simulink model "model6_3"  (R2025a)
settings: Solver=VariableStepAuto  StartTime=0.0  StopTime=100000  RelTol=1e-3
values from neighbouring files (symbols this model uses):
  Tf = 1    [domaci6_1.m]
settings Model: Creator=neso  LastModifiedBy=Nenad

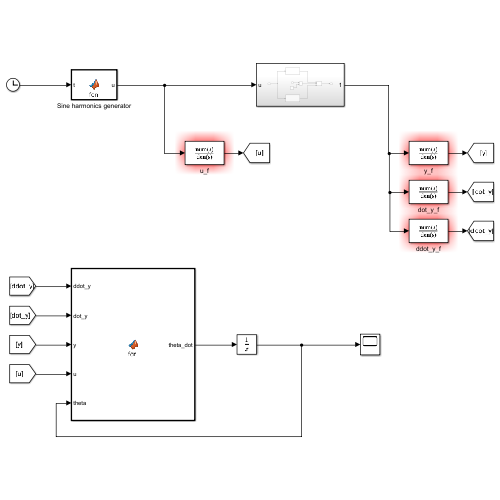
[thumbnail: Simulink's stored preview of the top-level diagram]
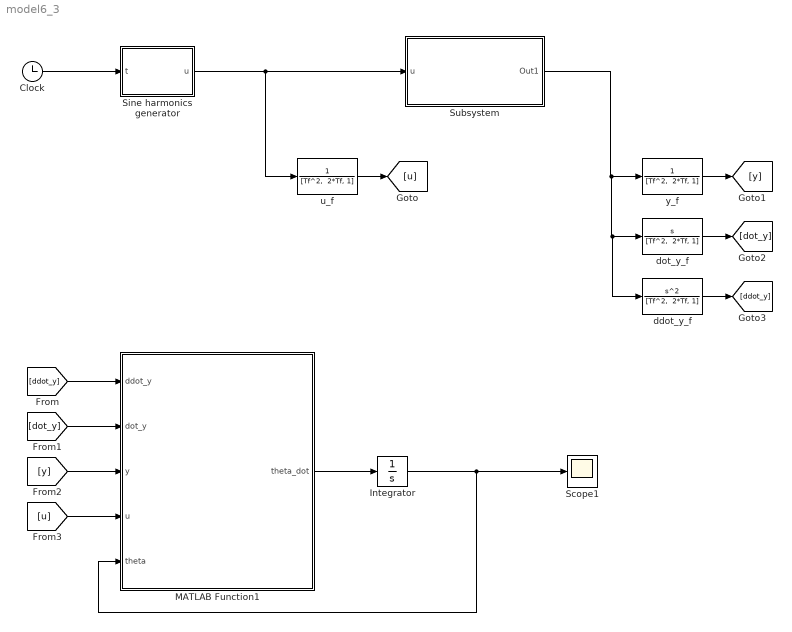
== system model6_3 ==
  Clock : Clock
  Integrator : Integrator  InitialCondition=[0; 0; 0]
  MATLAB Function1 : MATLAB Function  TreatAsAtomicUnit=on
  Scope1 : Scope
      settings: ActiveDisplayYMinimum=-1.07597  ActiveDisplayYMaximum=9.00844
  Sine harmonics generator : MATLAB Function  TreatAsAtomicUnit=on
  Subsystem : Subsystem
  ddot_y_f : TransferFcn  Numerator=[1, 0, 0]  Denominator="[Tf^2,  2*Tf, 1]"
  dot_y_f : TransferFcn  Numerator=[1, 0]  Denominator="[Tf^2,  2*Tf, 1]"
  u_f : TransferFcn  Denominator="[Tf^2,  2*Tf, 1]"
  y_f : TransferFcn  Denominator="[Tf^2,  2*Tf, 1]"
  wires:
  u_f/1 -> [u]
  y_f/1 -> [y]
  dot_y_f/1 -> [dot_y]
  ddot_y_f/1 -> [ddot_y]
  MATLAB Function1/1(theta_dot) -> Integrator/1
  [ddot_y] -> MATLAB Function1/1(ddot_y)
  [dot_y] -> MATLAB Function1/2(dot_y)
  [y] -> MATLAB Function1/3(y)
  [u] -> MATLAB Function1/4(u)
  Integrator/1 -> Scope1/1, MATLAB Function1/5(theta)
  Subsystem/1(Out1) -> ddot_y_f/1, dot_y_f/1, y_f/1
  Sine harmonics generator/1(u) -> u_f/1, Subsystem/1(u)
  Clock/1 -> Sine harmonics generator/1(t)

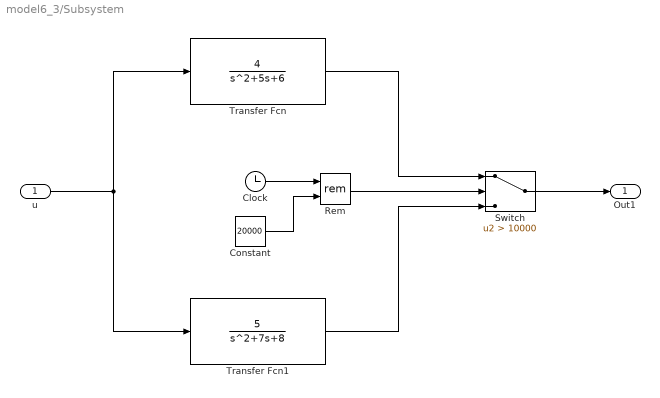
== system model6_3/Subsystem ==
  u : Inport
  Clock : Clock
  Constant : Constant  Value=20000
  Rem : Math  Operator=rem
  Switch : Switch  Criteria=u2 > Threshold  Threshold=10000  SaturateOnIntegerOverflow=off  InputSameDT=off
  Transfer Fcn : TransferFcn  Numerator=4  Denominator=[1, 5, 6]
  Transfer Fcn1 : TransferFcn  Numerator=5  Denominator=[1, 7, 8]
  Out1 : Outport
  wires:
  u/1 -> Transfer Fcn1/1, Transfer Fcn/1
  Transfer Fcn/1 -> Switch/1
  Transfer Fcn1/1 -> Switch/3
  Switch/1 -> Out1/1
  Clock/1 -> Rem/1
  Constant/1 -> Rem/2
  Rem/1 -> Switch/2

== matlab function model6_3/MATLAB Function1 ==
  data: ddot_y input; dot_y input; y input; u input; theta_dot output; theta input
function theta_dot = fcn(ddot_y, dot_y, y, u, theta)
    p = [-dot_y; -y; u];
    eta = ddot_y;

    G = 0.1 * eye(length(p), length(p));

    theta_dot = G * p * (eta - p' * theta);
end

== matlab function model6_3/Sine harmonics generator ==
  data: t input; u output
function u = fcn(t)
    u = 1;
    fmax = 20;
    for f = 1:fmax
        u = u + sin(2 * pi * f * t);
    end
end
